simulink model "uz_endat_interface_2025b"  (R2025b)
settings: Solver=FixedStepDiscrete  StartTime=0.0  StopTime=1.3e-3  RelTol=1e-3
values from neighbouring files (symbols this model uses):
  binary_or_gray = false    [uz_endat_interface_init.m]
  bit_sum = endat_encoder_bit_width_multi_turn+endat_encoder_bit_width_single_turn+endat_encoder_number_of_CRC_bits    [uz_endat_interface_init.m]
  delay_first_clk_on_off = true    [uz_endat_interface_init.m]
  endat_clk_divider = 25    [uz_endat_interface_init.m]
  endat_encoder_bit_width_multi_turn = uint32(12)    [uz_endat_interface_init.m]
  endat_encoder_bit_width_single_turn = uint32(25)    [uz_endat_interface_init.m]
  endat_encoder_number_of_CRC_bits = uint32(0)    [uz_endat_interface_init.m]
  f_ADC = 20e3    (= 20000)    [uz_endat_interface_init.m]
  f_clock = 100e6    (= 100000000)    [uz_endat_interface_init.m]
  t_ADC = 1/f_ADC    (= 5e-05)    [uz_endat_interface_init.m]
  t_clock = 1/f_clock    (= 1e-08)    [uz_endat_interface_init.m]
undefined symbols (not defined in the file or in its folder): PLL
libraries: simulink x37, hdlsllib x32, simulink_extras x14, spsSampleandHoldLib x1
(part 2 of 3)

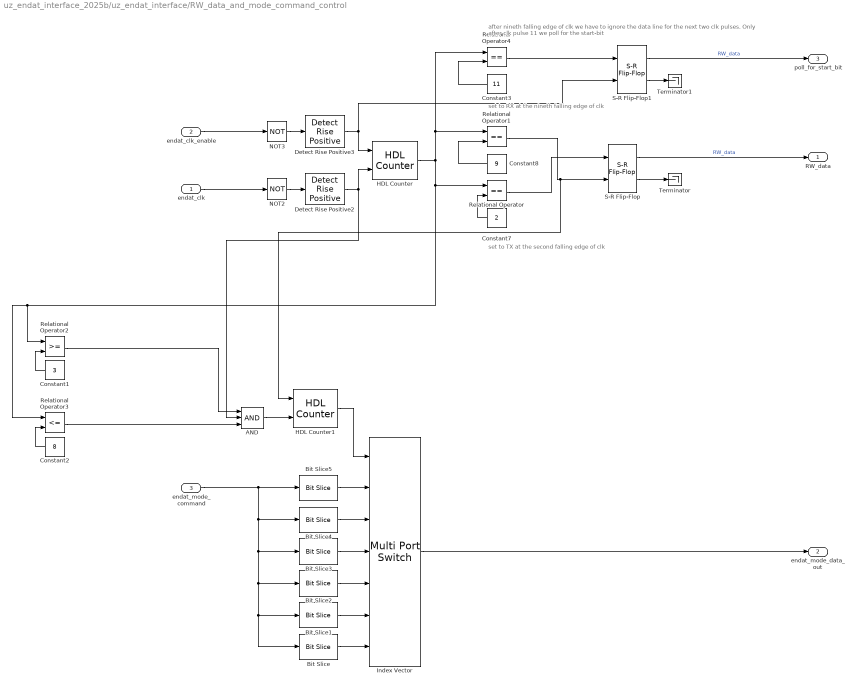
== system uz_endat_interface_2025b/uz_endat_interface/RW_data_and_mode_command_control ==
  note: set to TX at the second falling edge of clk
  note: set to RX at the nineth falling edge of clk
  note: after nineth falling edge of clk we have to ignore the data line for the next two clk pulses. Only after clk pulse 11 we poll for the start-bit
  endat_clk : Inport
  endat_clk_enable : Inport  Port=2
  endat_mode_command : Inport  Port=3
  AND : Logic  Inputs=3  IconShape=distinctive  AllPortsSameDT=off  OutDataTypeStr=boolean
  Bit Slice : hdlsllib/Logic and Bit Operations/Bit Slice  lidx=0  ridx=0
  Bit Slice1 : hdlsllib/Logic and Bit Operations/Bit Slice  lidx=1  ridx=1
  Bit Slice2 : hdlsllib/Logic and Bit Operations/Bit Slice  lidx=2  ridx=2
  Bit Slice3 : hdlsllib/Logic and Bit Operations/Bit Slice  lidx=3  ridx=3
  Bit Slice4 : hdlsllib/Logic and Bit Operations/Bit Slice  lidx=4  ridx=4
  Bit Slice5 : hdlsllib/Logic and Bit Operations/Bit Slice  lidx=5  ridx=5
  Constant1 : Constant  Value=3  OutDataTypeStr=uint8  SampleTime=-1
  Constant2 : Constant  Value=8  OutDataTypeStr=uint8  SampleTime=-1
  Constant3 : Constant  Value=11  OutDataTypeStr=uint8  SampleTime=-1
  Constant7 : Constant  Value=2  OutDataTypeStr=uint8  SampleTime=-1
  Constant8 : Constant  Value=9  OutDataTypeStr=uint8  SampleTime=-1
  Detect Rise Positive2 : simulink/Logic and Bit Operations/Detect Rise Positive  vinit=0  OutDataTypeStr=boolean
  Detect Rise Positive3 : simulink/Logic and Bit Operations/Detect Rise Positive  vinit=0  OutDataTypeStr=boolean
  HDL Counter : hdlsllib/Sources/HDL Counter  CountType=Free running  CountInit=0  CountStep=1  CountMax=25  CountFromType=Initial value  CountFrom=0  CountResetPort=on  CountLoadPort=off  CountEnbPort=on  CountDirPort=off  CountHitOutputPort=off  CountDataType=Unsigned  CountWordLen=8  CountFracLen=0  CountSampTime=1
  HDL Counter1 : hdlsllib/Sources/HDL Counter  CountType=Count limited  CountInit=0  CountStep=1  CountMax=5  CountFromType=Initial value  CountFrom=0  CountResetPort=on  CountLoadPort=off  CountEnbPort=on  CountDirPort=off  CountHitOutputPort=off  CountDataType=Unsigned  CountWordLen=8  CountFracLen=0  CountSampTime=1
  Index Vector : MultiPortSwitch  DataPortOrder=Zero-based contiguous  Inputs=6  zeroidx=on  SaturateOnIntegerOverflow=off  InputSameDT=off
  NOT2 : Logic  Operator=NOT  IconShape=distinctive  AllPortsSameDT=off  OutDataTypeStr=boolean
  NOT3 : Logic  Operator=NOT  IconShape=distinctive  AllPortsSameDT=off  OutDataTypeStr=boolean
  Relational Operator : RelationalOperator  Operator===  OutDataTypeStr=boolean  RndMeth=Simplest  InputSameDT=off
  Relational Operator1 : RelationalOperator  Operator===  OutDataTypeStr=boolean  RndMeth=Simplest  InputSameDT=off
  Relational Operator2 : RelationalOperator  OutDataTypeStr=boolean  RndMeth=Simplest  InputSameDT=off
  Relational Operator3 : RelationalOperator  Operator=<=  OutDataTypeStr=boolean  RndMeth=Simplest  InputSameDT=off
  Relational Operator4 : RelationalOperator  Operator===  OutDataTypeStr=boolean  RndMeth=Simplest  InputSameDT=off
  S-R Flip-Flop : simulink_extras/Flip Flops/S-R Flip-Flop  initial_condition=0
  S-R Flip-Flop1 : simulink_extras/Flip Flops/S-R Flip-Flop  initial_condition=0
  Terminator : Terminator
  Terminator1 : Terminator
  RW_data : Outport
  endat_mode_data_out : Outport  Port=2
  poll_for_start_bit : Outport  Port=3
  wires:
  Constant7/1 -> Relational Operator/2
  HDL Counter/1 -> Relational Operator2/1, Relational Operator3/1, Relational Operator/1, Relational Operator4/1, Relational Operator1/1
  endat_clk_enable/1 -> NOT3/1
  S-R Flip-Flop/2 -> Terminator/1
  Constant8/1 -> Relational Operator1/2
  NOT2/1 -> Detect Rise Positive2/1
  endat_clk/1 -> NOT2/1
  NOT3/1 -> Detect Rise Positive3/1
  S-R Flip-Flop/1 -> RW_data/1  "RW_data"
  Relational Operator/1 -> S-R Flip-Flop/1
  Detect Rise Positive3/1 -> HDL Counter/1, S-R Flip-Flop1/2
  Bit Slice/1 -> Index Vector/7
  Bit Slice3/1 -> Index Vector/4
  Bit Slice2/1 -> Index Vector/5
  Bit Slice1/1 -> Index Vector/6
  Bit Slice4/1 -> Index Vector/3
  Bit Slice5/1 -> Index Vector/2
  endat_mode_command/1 -> Bit Slice4/1, Bit Slice3/1, Bit Slice2/1, Bit Slice1/1, Bit Slice/1, Bit Slice5/1
  AND/1 -> HDL Counter1/2
  Constant1/1 -> Relational Operator2/2
  HDL Counter1/1 -> Index Vector/1
  Constant2/1 -> Relational Operator3/2
  Relational Operator1/1 -> HDL Counter1/1, S-R Flip-Flop/2
  Detect Rise Positive2/1 -> AND/2, HDL Counter/2
  Relational Operator2/1 -> AND/1
  Relational Operator3/1 -> AND/3
  Index Vector/1 -> endat_mode_data_out/1
  Constant3/1 -> Relational Operator4/2
  Relational Operator4/1 -> S-R Flip-Flop1/1
  S-R Flip-Flop1/1 -> poll_for_start_bit/1  "RW_data"
  S-R Flip-Flop1/2 -> Terminator1/1

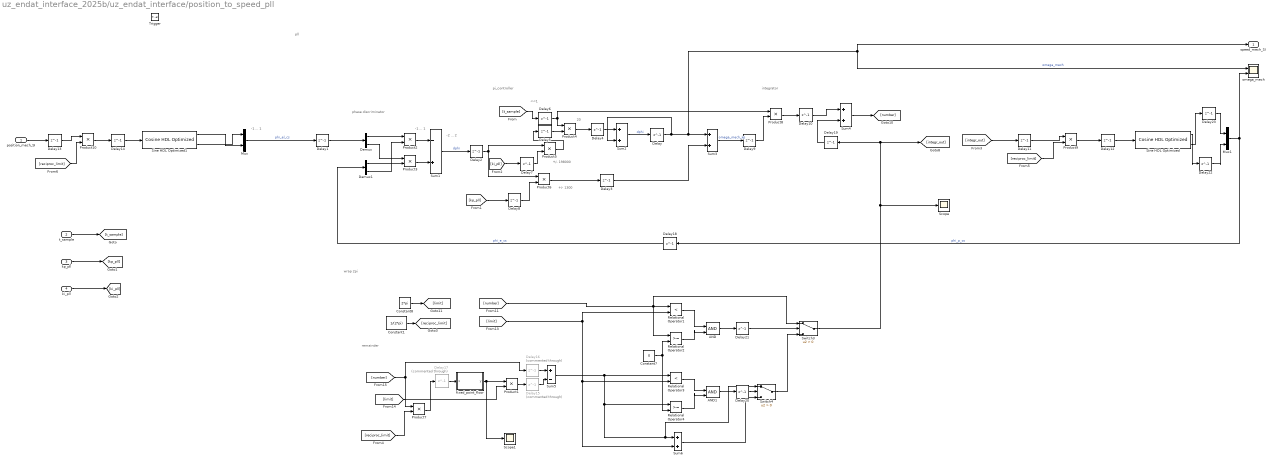
== system uz_endat_interface_2025b/uz_endat_interface/position_to_speed_pll ==
  note: remainder
  note: +/- 1300
  note: 20
  note: integrator
  note: -1 ... 1
  note: pll
  note: -1 ... 1
  note: phase discriminator
  note: <<1
  note: wrap 2pi
  note: -2 ... 2
  note: +/- 198000
  note: pi_controller
  position_mech_SI : Inport
  t_sample : Inport  Port=2
  kp_pll : Inport  Port=3
  ki_pll : Inport  Port=4
  Trigger : TriggerPort  VariantControl=(inherit)  InitialTriggerSignalState=zero
  AND : Logic  IconShape=distinctive  AllPortsSameDT=off  OutDataTypeStr=boolean
  AND1 : Logic  IconShape=distinctive  AllPortsSameDT=off  OutDataTypeStr=boolean
  Constant1 : Constant  Value=1/(2*pi)  OutDataTypeStr=fixdt(0,18,20)  SampleTime=-1
  Constant7 : Constant  Value=0  OutDataTypeStr=fixdt(0,27,24)  SampleTime=-1
  Constant8 : Constant  Value=2*pi  OutDataTypeStr=fixdt(0,18,15)  SampleTime=-1
  Delay{,19..23} (6 alike) : Delay  DelayLength=1
  Delay1 : Delay  DelayLength=1  InitialCondition=[1 0]
  Delay{2..14} (13 alike) : Delay  DelayLength=1  InitialCondition=0
  Delay15 : Delay  Commented=through  DelayLength=1  InitialCondition=0
  Delay16 : Delay  Commented=through  DelayLength=1  InitialCondition=0
  Delay17 : Delay  Commented=through  DelayLength=1  InitialCondition=0
  Delay18 : Delay  DelayLength=1  InitialCondition=[1 0]
  Demux : Demux  Outputs=2
  Demux1 : Demux  Outputs=2
  Mux : Mux  Inputs=2
  Mux1 : Mux  Inputs=2
  Product1 : Product  OutDataTypeStr=fixdt(1,27,23)
  Product10 : Product  OutDataTypeStr=fixdt(1,27,20)
  Product2 : Product  OutDataTypeStr=fixdt(1,27,25)
  Product3 : Product  OutDataTypeStr=fixdt(1,27,25)
  Product4 : Product  OutDataTypeStr=fixdt(1,27,20)
  Product5 : Product  OutDataTypeStr=fixdt(1,27,8)
  Product6 : Product  OutDataTypeStr=fixdt(1,27,14)
  Product7 : Product  OutDataTypeStr=fixdt(1,27,23)
  Product8 : Product  OutDataTypeStr=fixdt(1,27,26)
  Product9 : Product  OutDataTypeStr=fixdt(1,27,20)
  Relational Operator1 : RelationalOperator  Operator=<  OutDataTypeStr=boolean  RndMeth=Simplest  InputSameDT=off
  Relational Operator2 : RelationalOperator  OutDataTypeStr=boolean  RndMeth=Simplest  InputSameDT=off
  Relational Operator3 : RelationalOperator  Operator=<  OutDataTypeStr=boolean  RndMeth=Simplest  InputSameDT=off
  Relational Operator4 : RelationalOperator  OutDataTypeStr=boolean  RndMeth=Simplest  InputSameDT=off
  Scope : Scope
      settings: ActiveDisplayYMinimum=0.18141  ActiveDisplayYMaximum=6.96115  DataLoggingVariableName=ScopeData2
  Scope1 : Scope
      settings: ActiveDisplayYMinimum=-0.125  ActiveDisplayYMaximum=1.125  DataLoggingVariableName=ScopeData2
  Sine HDL Optimized : hdlsllib/Lookup Tables/Cosine HDL Optimized  OutputFormula=sin(2*pi*u) and cos(2*pi*u)  NumDataPoints=256  TableDataTypeStr=fixdt(0,26,20)  SimulateLUTROMDelay=off
      settings: LibrarySourceBlock=|
      | hdlsllib/Lookup
      | Tables/Sine
      | HDL Optimized
  Sine HDL Optimized1 : hdlsllib/Lookup Tables/Cosine HDL Optimized  OutputFormula=sin(2*pi*u) and cos(2*pi*u)  NumDataPoints=256  TableDataTypeStr=fixdt(0,26,20)  SimulateLUTROMDelay=off
      settings: LibrarySourceBlock=|
      | hdlsllib/Lookup
      | Tables/Sine
      | HDL Optimized
  Sum1 : Sum  Inputs=-+  AccumDataTypeStr=fixdt(1,27,24)
  Sum2 : Sum  OutDataTypeStr=fixdt(1,27,16)
  Sum3 : Sum  OutDataTypeStr=fixdt(1,27,14)
  Sum4 : Sum  OutDataTypeStr=fixdt(1,27,23)
  Sum5 : Sum  Inputs=+-  OutDataTypeStr=fixdt(1,27,23)
  Sum6 : Sum  OutDataTypeStr=fixdt(1,27,23)
  Switch3 : Switch  Criteria=u2 > Threshold  SaturateOnIntegerOverflow=off  InputSameDT=off
  Switch4 : Switch  Criteria=u2 > Threshold  SaturateOnIntegerOverflow=off  InputSameDT=off
  fixed_point_floor : MATLAB Function  TreatAsAtomicUnit=on
  omega_mech : Scope  NumInputPorts=2
      settings: ActiveDisplayYMinimum=-587.14492  ActiveDisplayYMaximum=357.65664
  speed_mech_SI : Outport  InitialOutput=[0]
  wires:
  Product2/1 -> Sum1/1
  Constant8/1 -> [limit]
  Delay19/1 -> Sum4/2
  Demux/1 -> Product2/1
  Mux1/1 -> omega_mech/2, Delay18/1  "phi_p_cs"
  [ki_pll] -> Delay7/1
  Sine HDL Optimized/2 -> Delay23/1
  Sum3/1 -> Delay9/1  "omega_mech_kp"
  Demux1/2 -> Product2/2
  Switch3/1 -> Scope/1, Delay19/1, [integr_out]
  Product3/1 -> Sum1/2
  Product4/1 -> Delay4/1
  Delay/1 -> speed_mech_SI/1, omega_mech/1, Sum3/1, Sum2/2  "omega_mech"
  Product8/1 -> Delay10/1
  [limit] -> Product1/2
  Switch4/1 -> Switch3/3
  [integr_out] -> Delay11/1
  Product1/1 -> Delay15/1
  Relational Operator3/1 -> AND1/1
  Product9/1 -> Delay12/1
  [number] -> Relational Operator2/1, Switch3/1, Relational Operator1/1
  Relational Operator2/1 -> AND/2
  Sum4/1 -> [number]
  Sum1/1 -> Delay2/1  "dphi"
  [limit] -> Relational Operator1/2, Sum6/2, Relational Operator3/2
  Product5/1 -> Delay5/1
  Product10/1 -> Delay14/1
  [number] -> Product7/1, Delay16/1
  Demux/2 -> Product3/1
  Delay6/1 -> Product4/1, Product8/1
  Demux1/1 -> Product3/2
  Delay18/1 -> Demux1/1  "phi_e_cs"
  Sine HDL Optimized/1 -> Delay22/1
  Mux/1 -> Delay1/1  "phi_el_cs"
  Relational Operator1/1 -> AND/1
  Product6/1 -> Delay3/1
  [kp_pll] -> Delay8/1
  AND/1 -> Delay21/1
  Sine HDL Optimized1/1 -> Mux/2
  Product7/1 -> Delay17/1
  Sum2/1 -> Delay/1  "dphi"
  Sum6/1 -> Switch4/3
  Sine HDL Optimized1/2 -> Mux/1
  Relational Operator4/1 -> AND1/2
  AND1/1 -> Delay20/1
  fixed_point_floor/1(y) -> Product1/1, Scope1/1
  position_mech_SI/1 -> Delay13/1
  Constant7/1 -> Relational Operator2/2, Relational Operator4/2
  t_sample/1 -> [t_sample]
  kp_pll/1 -> [kp_pll]
  ki_pll/1 -> [ki_pll]
  Delay1/1 -> Demux/1
  Delay2/1 -> Product5/1, Product6/1
  Delay3/1 -> Sum3/2
  Delay4/1 -> Sum2/1
  Delay5/1 -> Product4/2
  Delay7/1 -> Product5/2
  Delay8/1 -> Product6/2
  Delay9/1 -> Product8/2
  [t_sample] -> Delay6/1
  Delay10/1 -> Sum4/1
  Delay11/1 -> Product9/1
  Delay12/1 -> Sine HDL Optimized/1
  Delay13/1 -> Product10/1
  Delay14/1 -> Sine HDL Optimized1/1
  Delay15/1 -> Sum5/2
  Delay16/1 -> Sum5/1
  Delay17/1 -> fixed_point_floor/1(x)
  Sum5/1 -> Switch4/1, Sum6/1, Relational Operator4/1, Relational Operator3/1
  Constant1/1 -> [reciproc_limit]
  [reciproc_limit] -> Product7/2
  Delay20/1 -> Switch4/2
  Delay21/1 -> Switch3/2
  [reciproc_limit] -> Product9/2
  [reciproc_limit] -> Product10/2
  Delay22/1 -> Mux1/2
  Delay23/1 -> Mux1/1

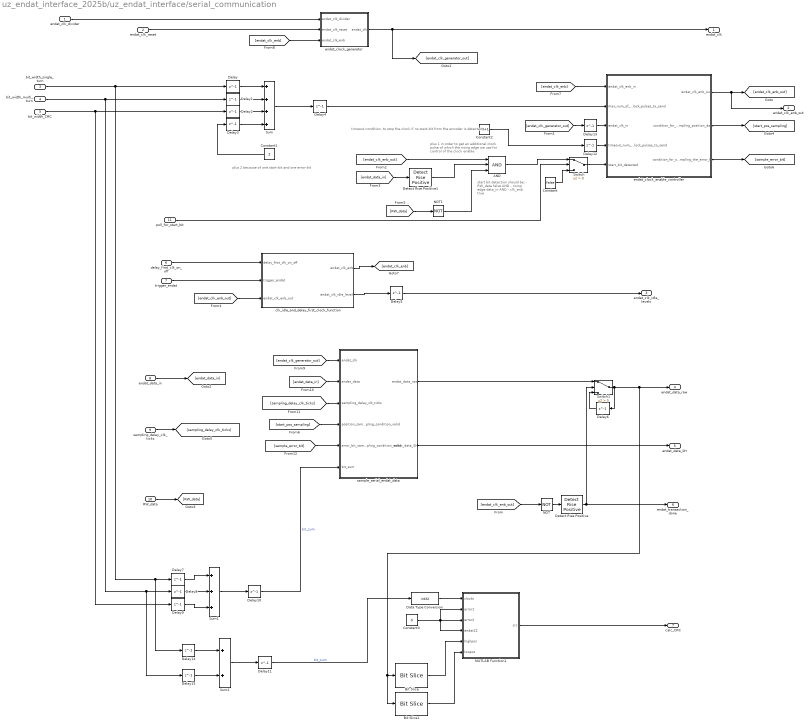
== system uz_endat_interface_2025b/uz_endat_interface/serial_communication ==
  note: plus 2 because of one start-bit and one error-bit
  note: timeout condition, to stop the clock if no start-bit from the encoder is detected
  note: plus 1 in order to get an additional clock pulse of which the rising edge we use for control of the clock enable
  note: start bit detection should be:
      | - RW_data false
      | AND
      | - rising edge data_in
      | AND
      | - clk_enb true
  endat_clk_divider : Inport
  endat_clk_reset : Inport  Port=2
  bit_width_single_turn : Inport  Port=3  OutDataTypeStr=uint32
  bit_width_multi_turn : Inport  Port=4  OutDataTypeStr=uint32
  bit_width_CRC : Inport  Port=5  OutDataTypeStr=uint32
  delay_first_clk_on_off : Inport  Port=6
  trigger_endat : Inport  Port=7
  endat_data_in : Inport  Port=8
  sampling_delay_clk_ticks : Inport  Port=9  OutDataTypeStr=uint32
  RW_data : Inport  Port=10
  poll_for_start_bit : Inport  Port=11
  AND : Logic  Inputs=3  IconShape=distinctive  AllPortsSameDT=off  OutDataTypeStr=boolean
  Bit Slice : hdlsllib/Logic and Bit Operations/Bit Slice  lidx=63  ridx=32
  Bit Slice1 : hdlsllib/Logic and Bit Operations/Bit Slice  lidx=31  ridx=0
  Constant : Constant  Value=false  SampleTime=-1
  Constant1 : Constant  Value=2  OutDataTypeStr=uint32  SampleTime=t_clock
  Constant2 : Constant  Value=70+1  OutDataTypeStr=uint32  SampleTime=t_clock
  Constant3 : Constant  Value=0  OutDataTypeStr=uint32  SampleTime=-1
  Data Type Conversion : DataTypeConversion  OutDataTypeStr=int32  SaturateOnIntegerOverflow=off  RndMeth=Floor
  Delay{,1..4,7..11,14..15} (12 alike) : Delay  DelayLength=1  InitialCondition=0
  Delay{5..6,12..13} (4 alike) : Delay  DelayLength=1
  Detect Rise Positive : simulink/Logic and Bit Operations/Detect Rise Positive  vinit=0  OutDataTypeStr=boolean
  Detect Rise Positive1 : simulink/Logic and Bit Operations/Detect Rise Positive  vinit=0  OutDataTypeStr=boolean
  MATLAB Function1 : MATLAB Function  TreatAsAtomicUnit=on
  NOT : Logic  Operator=NOT  IconShape=distinctive  AllPortsSameDT=off  OutDataTypeStr=boolean
  NOT1 : Logic  Operator=NOT  IconShape=distinctive  AllPortsSameDT=off  OutDataTypeStr=boolean
  Sum : Sum  Inputs=++++  OutDataTypeStr=uint32
  Sum1 : Sum  Inputs=+++  OutDataTypeStr=uint32
  Sum2 : Sum  OutDataTypeStr=uint32
  Switch : Switch  Criteria=u2 > Threshold  SaturateOnIntegerOverflow=off  InputSameDT=off
  Switch1 : Switch  Criteria=u2 > Threshold  SaturateOnIntegerOverflow=off  InputSameDT=off
  clk_idle_and_delay_first_clock_function : Subsystem
  endat_clock_enable_controller : Subsystem
  endat_clock_generator : Subsystem
  sample_serial_endat_data : Subsystem
  endat_clk : Outport
  endat_clk_enb_out : Outport  Port=2
  endat_clk_idle_levels : Outport  Port=3
  endat_data_raw : Outport  Port=4
  endat_data_SH : Outport  Port=5
  endat_transaction_done : Outport  Port=6
  calc_CRC : Outport  Port=7
  wires:
  Delay5/1 -> endat_clk_idle_levels/1
  [endat_clk_generator_out] -> sample_serial_endat_data/1(endat_clk)
  [endat_clk_enb] -> endat_clock_enable_controller/1(endat_clk_enb_in)
  endat_data_in/1 -> [endat_data_in]
  [endat_clk_generator_out] -> Delay13/1
  Detect Rise Positive/1 -> Switch1/2, endat_transaction_done/1
  Constant2/1 -> Delay12/1
  Delay12/1 -> endat_clock_enable_controller/4(timeout_num_of_clock_pulses_to_send)
  clk_idle_and_delay_first_clock_function/2(endat_clk_idle_levels) -> Delay5/1
  [endat_clk_enb_out] -> clk_idle_and_delay_first_clock_function/3(endat_clk_enb_out)
  endat_clock_enable_controller/1(endat_clk_enb_out) -> endat_clk_enb_out/1, [endat_clk_enb_out]
  Delay13/1 -> endat_clock_enable_controller/3(endat_clk_in)
  [endat_clk_enb] -> endat_clock_generator/3(endat_clk_enb)
  clk_idle_and_delay_first_clock_function/1(endat_clk_enb) -> [endat_clk_enb]
  sample_serial_endat_data/1(endat_data_raw) -> Switch1/1
  sample_serial_endat_data/2(endat_data_SH) -> endat_data_SH/1
  endat_clk_divider/1 -> endat_clock_generator/1(endat_clk_divider)
  endat_clk_reset/1 -> endat_clock_generator/2(endat_clk_reset)
  trigger_endat/1 -> clk_idle_and_delay_first_clock_function/2(trigger_endat)
  NOT/1 -> Detect Rise Positive/1
  [endat_clk_enb_out] -> NOT/1
  delay_first_clk_on_off/1 -> clk_idle_and_delay_first_clock_function/1(delay_first_clk_on_off)
  Constant1/1 -> Delay3/1
  [start_pos_sampling] -> sample_serial_endat_data/4(position_sampling_condition_valid)
  Sum/1 -> Delay4/1
  Switch/1 -> endat_clock_enable_controller/5(start_bit_detected)
  [endat_clk_enb_out] -> AND/1
  [endat_data_in] -> Detect Rise Positive1/1
  Detect Rise Positive1/1 -> AND/2
  RW_data/1 -> [RW_data]
  [RW_data] -> NOT1/1
  endat_clock_generator/1(endat_clk) -> endat_clk/1, [endat_clk_generator_out]
  NOT1/1 -> AND/3
  endat_clock_enable_controller/2(condition_for_start_sampling_position_data) -> [start_pos_sampling]
  [endat_data_in] -> sample_serial_endat_data/2(endat_data)
  sampling_delay_clk_ticks/1 -> [sampling_delay_clk_ticks]
  [sampling_delay_clk_ticks] -> sample_serial_endat_data/3(sampling_delay_clk_ticks)
  endat_clock_enable_controller/3(condition_for_sampling_the_error_bit) -> [sample_error_bit]
  [sample_error_bit] -> sample_serial_endat_data/5(error_bit_sampling_condition_valid)
  Delay/1 -> Sum/1
  Delay1/1 -> Sum/2
  Delay2/1 -> Sum/3
  Delay3/1 -> Sum/4
  Delay4/1 -> endat_clock_enable_controller/2(max_num_of_clock_pulses_to_send)
  AND/1 -> Switch/1
  poll_for_start_bit/1 -> Switch/2
  Constant/1 -> Switch/3
  Delay6/1 -> Switch1/3
  Switch1/1 -> Delay6/1, Bit Slice1/1, Bit Slice/1, endat_data_raw/1
  Delay7/1 -> Sum1/1
  Delay8/1 -> Sum1/2
  Sum1/1 -> Delay10/1
  bit_width_single_turn/1 -> Delay14/1, Delay7/1, Delay/1
  bit_width_CRC/1 -> Delay9/1, Delay2/1
  Delay9/1 -> Sum1/3
  bit_width_multi_turn/1 -> Delay15/1, Delay8/1, Delay1/1
  Delay10/1 -> sample_serial_endat_data/6(bit_sum)  "bit_sum"
  Delay15/1 -> Sum2/2
  Sum2/1 -> Delay11/1
  Delay14/1 -> Sum2/1
  Delay11/1 -> Data Type Conversion/1  "bit_sum"
  Constant3/1 -> MATLAB Function1/4(endat22), MATLAB Function1/3(error2), MATLAB Function1/2(error1)
  Bit Slice/1 -> MATLAB Function1/5(highpos)
  Bit Slice1/1 -> MATLAB Function1/6(lowpos)
  MATLAB Function1/1(crc) -> calc_CRC/1
  Data Type Conversion/1 -> MATLAB Function1/1(clocks)

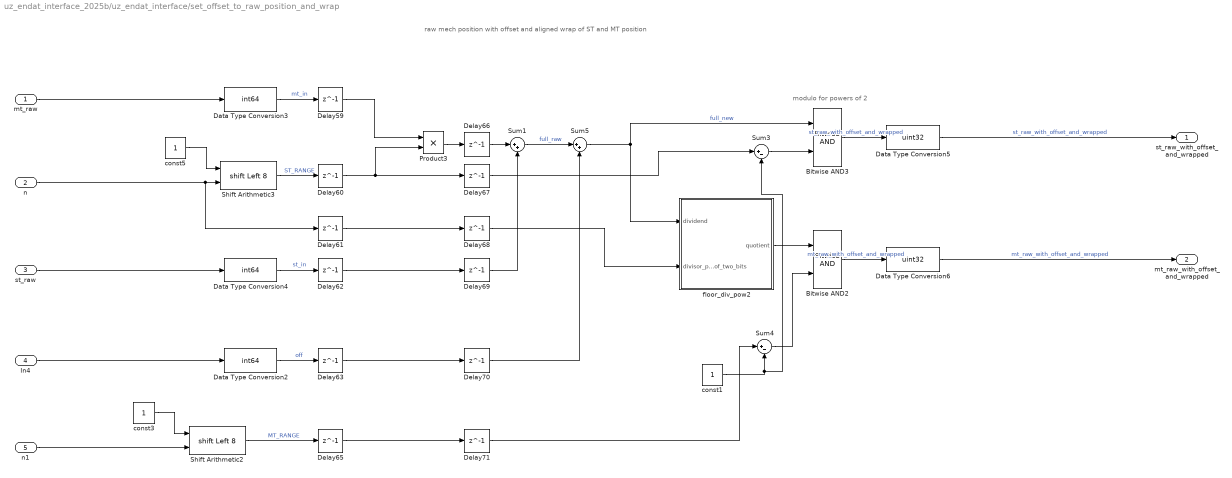
== system uz_endat_interface_2025b/uz_endat_interface/set_offset_to_raw_position_and_wrap ==
  note: raw mech position with offset and aligned wrap of ST and MT position
  note: modulo for powers of 2
  mt_raw : Inport
  n : Inport  Port=2
  st_raw : Inport  Port=3
  In4 : Inport  Port=4
  n1 : Inport  Port=5
  Bitwise AND2 : simulink/Logic and Bit Operations/Bitwise Operator  logicop=AND  UseBitMask=off  NumInputPorts=2  BitMask=bin2dec('11011001')  BitMaskRealWorld=Stored Integer
      settings: LibrarySourceBlock=|
      | simulink/Quick Insert/Logic and Bit
      | Operations/Bitwise AND
  Bitwise AND3 : simulink/Logic and Bit Operations/Bitwise Operator  logicop=AND  UseBitMask=off  NumInputPorts=2  BitMask=bin2dec('11011001')  BitMaskRealWorld=Stored Integer
      settings: LibrarySourceBlock=|
      | simulink/Quick Insert/Logic and Bit
      | Operations/Bitwise AND
  Data Type Conversion2 : DataTypeConversion  OutDataTypeStr=int64  SaturateOnIntegerOverflow=off  RndMeth=Floor
  Data Type Conversion3 : DataTypeConversion  OutDataTypeStr=int64  SaturateOnIntegerOverflow=off  RndMeth=Floor
  Data Type Conversion4 : DataTypeConversion  OutDataTypeStr=int64  SaturateOnIntegerOverflow=off  RndMeth=Floor
  Data Type Conversion5 : DataTypeConversion  OutDataTypeStr=uint32  SaturateOnIntegerOverflow=off  RndMeth=Floor
  Data Type Conversion6 : DataTypeConversion  OutDataTypeStr=uint32  SaturateOnIntegerOverflow=off  RndMeth=Floor
  Delay{59..63,65..71} (12 alike) : Delay  DelayLength=1  InitialCondition=0
  Product3 : Product  OutDataTypeStr=int64
  Shift Arithmetic2 : ArithShift  BitShiftNumberSource=Input port  BitShiftNumber=8  BitShiftDirection=Left
      settings: InputPortMap=u0,p1
  Shift Arithmetic3 : ArithShift  BitShiftNumberSource=Input port  BitShiftNumber=8  BitShiftDirection=Left
      settings: InputPortMap=u0,p1
  Sum1 : Sum  Inputs=|++  OutDataTypeStr=int64
  Sum3 : Sum  Inputs=|+-  OutDataTypeStr=int64
  Sum4 : Sum  Inputs=|+-  OutDataTypeStr=int64
  Sum5 : Sum  Inputs=|++  OutDataTypeStr=int64
  const1 : Constant  OutDataTypeStr=int64  SampleTime=t_clock
  const3 : Constant  OutDataTypeStr=int64  SampleTime=t_clock
  const5 : Constant  OutDataTypeStr=int64  SampleTime=t_clock
  floor_div_pow2 : Subsystem
  st_raw_with_offset_and_wrapped : Outport
  mt_raw_with_offset_and_wrapped : Outport  Port=2
  wires:
  mt_raw/1 -> Data Type Conversion3/1
  Delay62/1 -> Delay69/1
  Delay60/1 -> Product3/2, Delay67/1
  Data Type Conversion2/1 -> Delay63/1  "off"
  Data Type Conversion4/1 -> Delay62/1  "st_in"
  Delay70/1 -> Sum5/2
  Data Type Conversion3/1 -> Delay59/1  "mt_in"
  const1/1 -> Sum3/2, Sum4/2
  Delay68/1 -> floor_div_pow2/2(divisor_power_of_two_bits)
  Sum1/1 -> Sum5/1  "full_raw"
  Sum5/1 -> Bitwise AND3/1, floor_div_pow2/1(dividend)  "full_new"
  Product3/1 -> Delay66/1
  n/1 -> Delay61/1, Shift Arithmetic3/2
  Shift Arithmetic2/1 -> Delay65/1  "MT_RANGE"
  floor_div_pow2/1(quotient) -> Bitwise AND2/1
  Delay63/1 -> Delay70/1
  Bitwise AND3/1 -> Data Type Conversion5/1  "st_raw_with_offset_and_wrapped"
  Delay66/1 -> Sum1/1
  const5/1 -> Shift Arithmetic3/1
  const3/1 -> Shift Arithmetic2/1
  Bitwise AND2/1 -> Data Type Conversion6/1  "mt_raw_with_offset_and_wrapped"
  Delay71/1 -> Sum4/1
  Sum4/1 -> Bitwise AND2/2
  Shift Arithmetic3/1 -> Delay60/1  "ST_RANGE"
  st_raw/1 -> Data Type Conversion4/1
  Sum3/1 -> Bitwise AND3/2
  Delay61/1 -> Delay68/1
  Data Type Conversion6/1 -> mt_raw_with_offset_and_wrapped/1  "mt_raw_with_offset_and_wrapped"
  Delay65/1 -> Delay71/1
  Delay69/1 -> Sum1/2
  Delay67/1 -> Sum3/1
  Delay59/1 -> Product3/1
  In4/1 -> Data Type Conversion2/1
  n1/1 -> Shift Arithmetic2/2
  Data Type Conversion5/1 -> st_raw_with_offset_and_wrapped/1  "st_raw_with_offset_and_wrapped"

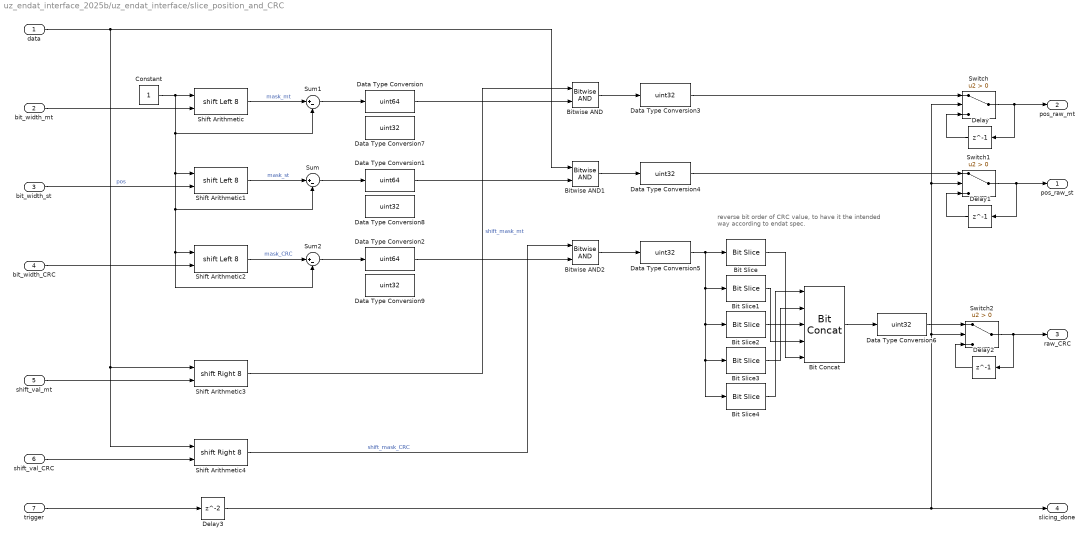
== system uz_endat_interface_2025b/uz_endat_interface/slice_position_and_CRC ==
  note: reverse bit order of CRC value, to have it
      | the intended way according to endat spec.
  data : Inport
  bit_width_mt : Inport  Port=2
  bit_width_st : Inport  Port=3
  bit_width_CRC : Inport  Port=4
  shift_val_mt : Inport  Port=5
  shift_val_CRC : Inport  Port=6
  trigger : Inport  Port=7
  Bit Concat : hdlsllib/Logic and Bit Operations/Bit Concat  numInputs=5
  Bit Slice : hdlsllib/Logic and Bit Operations/Bit Slice  lidx=4  ridx=4
  Bit Slice1 : hdlsllib/Logic and Bit Operations/Bit Slice  lidx=3  ridx=3
  Bit Slice2 : hdlsllib/Logic and Bit Operations/Bit Slice  lidx=2  ridx=2
  Bit Slice3 : hdlsllib/Logic and Bit Operations/Bit Slice  lidx=1  ridx=1
  Bit Slice4 : hdlsllib/Logic and Bit Operations/Bit Slice  lidx=0  ridx=0
  Bitwise AND : simulink/Logic and Bit Operations/Bitwise Operator  logicop=AND  UseBitMask=off  NumInputPorts=2  BitMask=bin2dec('11011001')  BitMaskRealWorld=Stored Integer
      settings: LibrarySourceBlock=|
      | simulink/Quick Insert/Logic and Bit
      | Operations/Bitwise AND
  Bitwise AND1 : simulink/Logic and Bit Operations/Bitwise Operator  logicop=AND  UseBitMask=off  NumInputPorts=2  BitMask=bin2dec('11011001')  BitMaskRealWorld=Stored Integer
      settings: LibrarySourceBlock=|
      | simulink/Quick Insert/Logic and Bit
      | Operations/Bitwise AND
  Bitwise AND2 : simulink/Logic and Bit Operations/Bitwise Operator  logicop=AND  UseBitMask=off  NumInputPorts=2  BitMask=bin2dec('11011001')  BitMaskRealWorld=Stored Integer
      settings: LibrarySourceBlock=|
      | simulink/Quick Insert/Logic and Bit
      | Operations/Bitwise AND
  Constant : Constant  OutDataTypeStr=uint32  SampleTime=t_clock
  Data Type Conversion : DataTypeConversion  OutDataTypeStr=uint64  SaturateOnIntegerOverflow=off  RndMeth=Floor
  Data Type Conversion1 : DataTypeConversion  OutDataTypeStr=uint64  SaturateOnIntegerOverflow=off  RndMeth=Floor
  Data Type Conversion2 : DataTypeConversion  OutDataTypeStr=uint64  SaturateOnIntegerOverflow=off  RndMeth=Floor
  Data Type Conversion{3..9} (7 alike) : DataTypeConversion  OutDataTypeStr=uint32  SaturateOnIntegerOverflow=off  RndMeth=Floor
  Delay : Delay  DelayLength=1
  Delay1 : Delay  DelayLength=1
  Delay2 : Delay  DelayLength=1
  Delay3 : Delay
  Shift Arithmetic : ArithShift  BitShiftNumberSource=Input port  BitShiftNumber=8  BitShiftDirection=Left
      settings: InputPortMap=u0,p1
  Shift Arithmetic1 : ArithShift  BitShiftNumberSource=Input port  BitShiftNumber=8  BitShiftDirection=Left
      settings: InputPortMap=u0,p1
  Shift Arithmetic2 : ArithShift  BitShiftNumberSource=Input port  BitShiftNumber=8  BitShiftDirection=Left
      settings: InputPortMap=u0,p1
  Shift Arithmetic3 : ArithShift  BitShiftNumberSource=Input port  BitShiftNumber=8  BitShiftDirection=Right
      settings: InputPortMap=u0,p1
  Shift Arithmetic4 : ArithShift  BitShiftNumberSource=Input port  BitShiftNumber=8  BitShiftDirection=Right
      settings: InputPortMap=u0,p1
  Sum : Sum  Inputs=|+-  OutDataTypeStr=uint32
  Sum1 : Sum  Inputs=|+-  OutDataTypeStr=uint32
  Sum2 : Sum  Inputs=|+-  OutDataTypeStr=uint32
  Switch : Switch  Criteria=u2 > Threshold  SaturateOnIntegerOverflow=off  InputSameDT=off
  Switch1 : Switch  Criteria=u2 > Threshold  SaturateOnIntegerOverflow=off  InputSameDT=off
  Switch2 : Switch  Criteria=u2 > Threshold  SaturateOnIntegerOverflow=off  InputSameDT=off
  pos_raw_st : Outport
  pos_raw_mt : Outport  Port=2
  raw_CRC : Outport  Port=3
  slicing_done : Outport  Port=4
  wires:
  Constant/1 -> Shift Arithmetic/1, Sum1/2, Shift Arithmetic1/1, Shift Arithmetic2/1, Sum2/2, Sum/2
  Shift Arithmetic1/1 -> Sum/1  "mask_st"
  bit_width_st/1 -> Shift Arithmetic1/2  "pos"
  Sum/1 -> Data Type Conversion1/1
  bit_width_mt/1 -> Shift Arithmetic/2
  bit_width_CRC/1 -> Shift Arithmetic2/2
  Shift Arithmetic/1 -> Sum1/1  "mask_mt"
  Shift Arithmetic2/1 -> Sum2/1  "mask_CRC"
  Sum1/1 -> Data Type Conversion/1
  Sum2/1 -> Data Type Conversion2/1
  Bitwise AND2/1 -> Data Type Conversion5/1
  data/1 -> Bitwise AND1/1, Shift Arithmetic4/1, Shift Arithmetic3/1
  Bitwise AND/1 -> Data Type Conversion3/1
  Bitwise AND1/1 -> Data Type Conversion4/1
  shift_val_mt/1 -> Shift Arithmetic3/2
  shift_val_CRC/1 -> Shift Arithmetic4/2
  Shift Arithmetic3/1 -> Bitwise AND/1  "shift_mask_mt"
  Data Type Conversion1/1 -> Bitwise AND1/2
  Data Type Conversion/1 -> Bitwise AND/2
  Data Type Conversion2/1 -> Bitwise AND2/2
  Shift Arithmetic4/1 -> Bitwise AND2/1  "shift_mask_CRC"
  Data Type Conversion3/1 -> Switch/1
  Data Type Conversion4/1 -> Switch1/1
  Data Type Conversion5/1 -> Bit Slice4/1, Bit Slice3/1, Bit Slice2/1, Bit Slice1/1, Bit Slice/1
  Switch/1 -> Delay/1, pos_raw_mt/1
  Switch1/1 -> Delay1/1, pos_raw_st/1
  Switch2/1 -> Delay2/1, raw_CRC/1
  Delay2/1 -> Switch2/3
  Delay1/1 -> Switch1/3
  Delay/1 -> Switch/3
  trigger/1 -> Delay3/1
  Delay3/1 -> slicing_done/1, Switch1/2, Switch/2, Switch2/2
  Bit Slice2/1 -> Bit Concat/3
  Bit Slice/1 -> Bit Concat/5
  Bit Slice4/1 -> Bit Concat/1
  Bit Slice1/1 -> Bit Concat/4
  Bit Slice3/1 -> Bit Concat/2
  Bit Concat/1 -> Data Type Conversion6/1
  Data Type Conversion6/1 -> Switch2/1

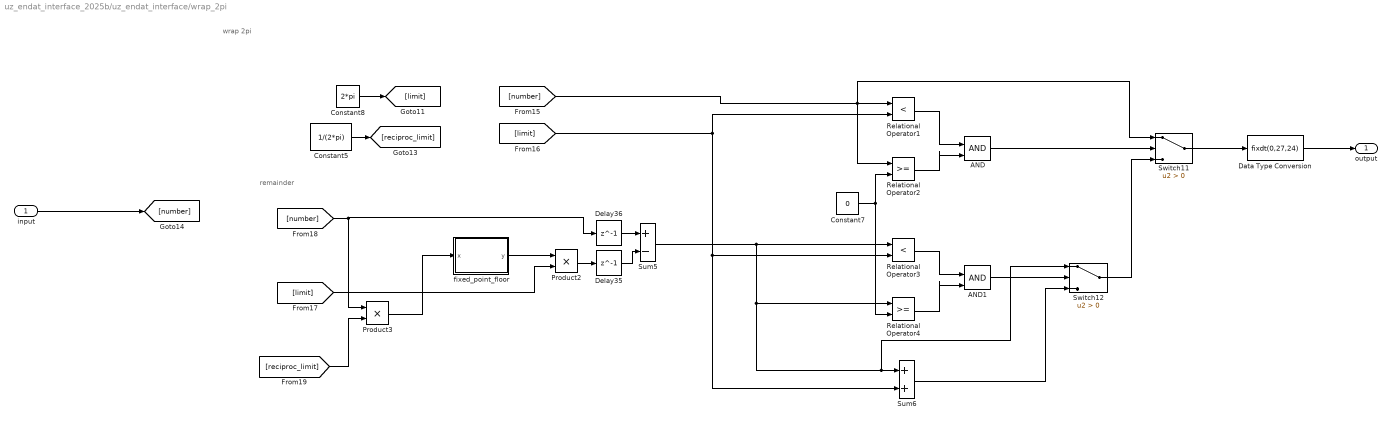
== system uz_endat_interface_2025b/uz_endat_interface/wrap_2pi ==
  note: wrap 2pi
  note: remainder
  input : Inport
  AND : Logic  IconShape=distinctive  AllPortsSameDT=off  OutDataTypeStr=boolean
  AND1 : Logic  IconShape=distinctive  AllPortsSameDT=off  OutDataTypeStr=boolean
  Constant5 : Constant  Value=1/(2*pi)  OutDataTypeStr=fixdt(0,18,20)  SampleTime=-1
  Constant7 : Constant  Value=0  OutDataTypeStr=fixdt(0,27,24)  SampleTime=-1
  Constant8 : Constant  Value=2*pi  OutDataTypeStr=fixdt(0,18,15)  SampleTime=-1
  Data Type Conversion : DataTypeConversion  OutDataTypeStr=fixdt(0,27,24)  SaturateOnIntegerOverflow=off  RndMeth=Floor
  Delay35 : Delay  DelayLength=1  InitialCondition=0
  Delay36 : Delay  DelayLength=1  InitialCondition=0
  Product2 : Product  OutDataTypeStr=fixdt(0,27,24)
  Product3 : Product  OutDataTypeStr=fixdt(0,27,24)
  Relational Operator1 : RelationalOperator  Operator=<  OutDataTypeStr=boolean  RndMeth=Simplest  InputSameDT=off
  Relational Operator2 : RelationalOperator  OutDataTypeStr=boolean  RndMeth=Simplest  InputSameDT=off
  Relational Operator3 : RelationalOperator  Operator=<  OutDataTypeStr=boolean  RndMeth=Simplest  InputSameDT=off
  Relational Operator4 : RelationalOperator  OutDataTypeStr=boolean  RndMeth=Simplest  InputSameDT=off
  Sum5 : Sum  Inputs=+-  OutDataTypeStr=fixdt(0,27,24)
  Sum6 : Sum  OutDataTypeStr=fixdt(0,27,24)
  Switch11 : Switch  Criteria=u2 > Threshold  SaturateOnIntegerOverflow=off  InputSameDT=off
  Switch12 : Switch  Criteria=u2 > Threshold  SaturateOnIntegerOverflow=off  InputSameDT=off
  fixed_point_floor : MATLAB Function  TreatAsAtomicUnit=on
  output : Outport
  wires:
  [number] -> Relational Operator2/1, Switch11/1, Relational Operator1/1
  Product2/1 -> Delay35/1
  [number] -> Delay36/1, Product3/1
  [reciproc_limit] -> Product3/2
  Delay35/1 -> Sum5/2
  Switch11/1 -> Data Type Conversion/1
  Relational Operator2/1 -> AND/2
  AND/1 -> Switch11/2
  Sum5/1 -> Switch12/1, Sum6/1, Relational Operator4/1, Relational Operator3/1
  Relational Operator1/1 -> AND/1
  [limit] -> Relational Operator1/2, Sum6/2, Relational Operator3/2
  Sum6/1 -> Switch12/3
  Delay36/1 -> Sum5/1
  Constant7/1 -> Relational Operator2/2, Relational Operator4/2
  Constant5/1 -> [reciproc_limit]
  Relational Operator4/1 -> AND1/2
  fixed_point_floor/1(y) -> Product2/1
  Product3/1 -> fixed_point_floor/1(x)
  AND1/1 -> Switch12/2
  [limit] -> Product2/2
  input/1 -> [number]
  Relational Operator3/1 -> AND1/1
  Switch12/1 -> Switch11/3
  Constant8/1 -> [limit]
  Data Type Conversion/1 -> output/1

== system uz_endat_interface_2025b/uz_endat_interface/Gray_code_to_binary/gray_to_bin ==
  gray : Inport
  enb : Inport  Port=2
  Bitwise OR1 : simulink/Logic and Bit Operations/Bitwise Operator  logicop=XOR  UseBitMask=off  NumInputPorts=2  BitMask=bin2dec('11011001')  BitMaskRealWorld=Stored Integer
      settings: LibrarySourceBlock=|
      | simulink/Quick Insert/Logic and Bit
      | Operations/Bitwise OR
  Constant4 : Constant  Value=63  OutMin=0  OutMax=63  OutDataTypeStr=fixdt(0,6)  SampleTime=t_clock
  Delay : Delay  DelayLength=1
  Delay2 : Delay  DelayLength=1
  Detect Rise Positive : simulink/Logic and Bit Operations/Detect Rise Positive  vinit=0  OutDataTypeStr=boolean
  Detect Rise Positive1 : simulink/Logic and Bit Operations/Detect Rise Positive  vinit=0  OutDataTypeStr=boolean
  HDL Counter : hdlsllib/Sources/HDL Counter  CountType=Count limited  CountInit=0  CountStep=1  CountMax=63  CountFromType=Initial value  CountFrom=0  CountResetPort=on  CountLoadPort=off  CountEnbPort=on  CountDirPort=off  CountHitOutputPort=off  CountDataType=Unsigned  CountWordLen=6  CountFracLen=0  CountSampTime=t_clock
  OR : Logic  Operator=OR  IconShape=distinctive  AllPortsSameDT=off  OutDataTypeStr=boolean
  Relational Operator2 : RelationalOperator  Operator===  OutDataTypeStr=boolean  RndMeth=Simplest  InputSameDT=off
  S-R Flip-Flop : simulink_extras/Flip Flops/S-R Flip-Flop  initial_condition=0
  Shift Arithmetic : ArithShift  BitShiftNumberSource=Input port  BitShiftNumber=8  BitShiftDirection=Right
      settings: InputPortMap=u0,p1
  Switch : Switch  Criteria=u2 > Threshold  SaturateOnIntegerOverflow=off  InputSameDT=off
  Switch3 : Switch  Criteria=u2 > Threshold  SaturateOnIntegerOverflow=off  InputSameDT=off
  binary_out : Outport
  wires:
  gray/1 -> Shift Arithmetic/1, Switch/1
  HDL Counter/1 -> Relational Operator2/1, Shift Arithmetic/2  "count"
  Switch3/1 -> binary_out/1, Delay2/1
  Constant4/1 -> Relational Operator2/2
  Delay2/1 -> Switch3/3
  Shift Arithmetic/1 -> Bitwise OR1/2  "shift_val"
  Relational Operator2/1 -> Detect Rise Positive/1
  enb/1 -> S-R Flip-Flop/1, OR/1, Detect Rise Positive1/1
  S-R Flip-Flop/1 -> HDL Counter/2
  Detect Rise Positive/1 -> Switch3/2, S-R Flip-Flop/2
  OR/1 -> HDL Counter/1
  S-R Flip-Flop/2 -> OR/2
  Detect Rise Positive1/1 -> Switch/2
  Switch/1 -> Bitwise OR1/1
  Bitwise OR1/1 -> Switch3/1, Delay/1  "binary_tmp"
  Delay/1 -> Switch/3

== system uz_endat_interface_2025b/uz_endat_interface/serial_communication/clk_idle_and_delay_first_clock_function ==
  note: 194 equals 2.0µs
  note: set idle level of clk to high (one),
      | and pull low when trigger_endat_read
      | is triggered
  delay_first_clk_on_off : Inport
  trigger_endat : Inport  Port=2
  endat_clk_enb_out : Inport  Port=3
  Constant4 : Constant  Value=0  OutDataTypeStr=boolean  SampleTime=t_clock
  Constant5 : Constant  OutDataTypeStr=boolean  SampleTime=t_clock
  Delay : Delay  DelayLength=194
  Delay1 : Delay  DelayLength=1
  Detect Rise Positive2 : simulink/Logic and Bit Operations/Detect Rise Positive  vinit=0  OutDataTypeStr=boolean
  NOT : Logic  Operator=NOT  IconShape=distinctive  AllPortsSameDT=off  OutDataTypeStr=boolean
  S-R Flip-Flop : simulink_extras/Flip Flops/S-R Flip-Flop  initial_condition=0
  Switch : Switch  Criteria=u2 > Threshold  SaturateOnIntegerOverflow=off  InputSameDT=off
  Switch3 : Switch  Criteria=u2 > Threshold  SaturateOnIntegerOverflow=off  InputSameDT=off
  Switch4 : Switch  Criteria=u2 > Threshold  SaturateOnIntegerOverflow=off  InputSameDT=off
  Terminator : Terminator
  endat_clk_enb : Outport
  endat_clk_idle_levels : Outport  Port=2
  wires:
  S-R Flip-Flop/2 -> Terminator/1
  Constant5/1 -> Switch/3
  Constant4/1 -> Switch/1
  NOT/1 -> Detect Rise Positive2/1
  Detect Rise Positive2/1 -> S-R Flip-Flop/2
  endat_clk_enb_out/1 -> NOT/1
  Switch/1 -> endat_clk_idle_levels/1
  trigger_endat/1 -> S-R Flip-Flop/1
  Delay/1 -> Switch4/1
  delay_first_clk_on_off/1 -> Switch3/2
  S-R Flip-Flop/1 -> Switch/2, Delay/1, Delay1/1
  Switch4/1 -> Switch3/1
  Delay1/1 -> Switch3/3, Switch4/3, Switch4/2
  Switch3/1 -> endat_clk_enb/1

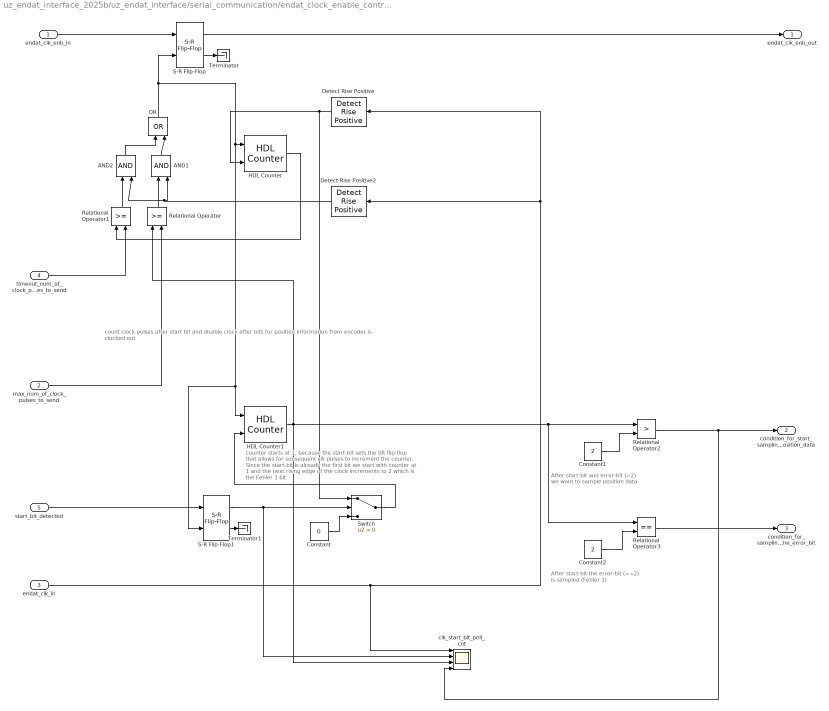
== system uz_endat_interface_2025b/uz_endat_interface/serial_communication/endat_clock_enable_controller ==
  note: counter starts at 1, because the start-bit sets the SR flip-flop that allows for subsequent clk pulses to increment the counter. Since the start-bit is already the first bit we start with counter at 1 and the next rising edge of the clock increments to 2 which is the Fehler 1 bit
  note: After start-bit and error-bit (=2)
      | we want to sample position data
  note: count clock pulses after start bit and disable clock after bits for position information from encoder is clocked out
  note: After start-bit the error-bit (==2)
      | is sampled (Fehler 1)
  endat_clk_enb_in : Inport
  max_num_of_clock_pulses_to_send : Inport  Port=2
  endat_clk_in : Inport  Port=3
  timeout_num_of_clock_pulses_to_send : Inport  Port=4
  start_bit_detected : Inport  Port=5
  AND1 : Logic  IconShape=distinctive  AllPortsSameDT=off  OutDataTypeStr=boolean
  AND2 : Logic  IconShape=distinctive  AllPortsSameDT=off  OutDataTypeStr=boolean
  Constant : Constant  Value=0  OutDataTypeStr=boolean  SampleTime=-1
  Constant1 : Constant  Value=2  OutDataTypeStr=uint8  SampleTime=-1
  Constant2 : Constant  Value=2  OutDataTypeStr=uint8  SampleTime=-1
  Detect Rise Positive : simulink/Logic and Bit Operations/Detect Rise Positive  vinit=0  OutDataTypeStr=boolean
  Detect Rise Positive2 : simulink/Logic and Bit Operations/Detect Rise Positive  vinit=0  OutDataTypeStr=boolean
  HDL Counter : hdlsllib/Sources/HDL Counter  CountType=Free running  CountInit=0  CountStep=1  CountMax=25  CountFromType=Initial value  CountFrom=0  CountResetPort=on  CountLoadPort=off  CountEnbPort=on  CountDirPort=off  CountHitOutputPort=off  CountDataType=Unsigned  CountWordLen=8  CountFracLen=0  CountSampTime=1
  HDL Counter1 : hdlsllib/Sources/HDL Counter  CountType=Free running  CountInit=1  CountStep=1  CountMax=25  CountFromType=Initial value  CountFrom=1  CountResetPort=on  CountLoadPort=off  CountEnbPort=on  CountDirPort=off  CountHitOutputPort=off  CountDataType=Unsigned  CountWordLen=8  CountFracLen=0  CountSampTime=1
  OR : Logic  Operator=OR  IconShape=distinctive  AllPortsSameDT=off  OutDataTypeStr=boolean
  Relational Operator : RelationalOperator  OutDataTypeStr=boolean  RndMeth=Simplest  InputSameDT=off
  Relational Operator1 : RelationalOperator  OutDataTypeStr=boolean  RndMeth=Simplest  InputSameDT=off
  Relational Operator2 : RelationalOperator  Operator=>  OutDataTypeStr=boolean  RndMeth=Simplest  InputSameDT=off
  Relational Operator3 : RelationalOperator  Operator===  OutDataTypeStr=boolean  RndMeth=Simplest  InputSameDT=off
  S-R Flip-Flop : simulink_extras/Flip Flops/S-R Flip-Flop  initial_condition=0
  S-R Flip-Flop1 : simulink_extras/Flip Flops/S-R Flip-Flop  initial_condition=0
  Switch : Switch  Criteria=u2 > Threshold  SaturateOnIntegerOverflow=off  InputSameDT=off
  Terminator : Terminator
  Terminator1 : Terminator
  clk_start_bit_poll_cnt : Scope  NumInputPorts=4
      settings: ActiveDisplayYMinimum=-0.125  ActiveDisplayYMaximum=1.125  DataLoggingVariableName=ScopeData3
  endat_clk_enb_out : Outport
  condition_for_start_sampling_position_data : Outport  Port=2
  condition_for_sampling_the_error_bit : Outport  Port=3
  wires:
  HDL Counter/1 -> Relational Operator1/1
  max_num_of_clock_pulses_to_send/1 -> Relational Operator/2
  S-R Flip-Flop/2 -> Terminator/1
  Relational Operator/1 -> AND1/1
  Detect Rise Positive/1 -> Switch/1, HDL Counter/2
  endat_clk_in/1 -> clk_start_bit_poll_cnt/1, Detect Rise Positive/1, Detect Rise Positive2/1
  S-R Flip-Flop/1 -> endat_clk_enb_out/1
  Detect Rise Positive2/1 -> AND2/2, AND1/2
  endat_clk_enb_in/1 -> S-R Flip-Flop/1
  AND1/1 -> OR/2
  Relational Operator1/1 -> AND2/1
  timeout_num_of_clock_pulses_to_send/1 -> Relational Operator1/2
  AND2/1 -> OR/1
  HDL Counter1/1 -> clk_start_bit_poll_cnt/3, Relational Operator3/1, Relational Operator2/1, Relational Operator/1
  OR/1 -> S-R Flip-Flop/2, S-R Flip-Flop1/2, HDL Counter1/1, HDL Counter/1
  start_bit_detected/1 -> S-R Flip-Flop1/1
  S-R Flip-Flop1/1 -> clk_start_bit_poll_cnt/2, Switch/2
  Constant/1 -> Switch/3
  Switch/1 -> HDL Counter1/2
  S-R Flip-Flop1/2 -> Terminator1/1
  Constant1/1 -> Relational Operator2/2
  Relational Operator2/1 -> clk_start_bit_poll_cnt/4, condition_for_start_sampling_position_data/1
  Constant2/1 -> Relational Operator3/2
  Relational Operator3/1 -> condition_for_sampling_the_error_bit/1

== system uz_endat_interface_2025b/uz_endat_interface/serial_communication/endat_clock_generator ==
  endat_clk_divider : Inport
  endat_clk_reset : Inport  Port=2
  endat_clk_enb : Inport  Port=3
  AND : Logic  IconShape=distinctive  AllPortsSameDT=off  OutDataTypeStr=boolean
  AND1 : Logic  IconShape=distinctive  AllPortsSameDT=off  OutDataTypeStr=boolean
  Constant : Constant  OutDataTypeStr=uint16  SampleTime=t_clock
  Data Type Conversion : DataTypeConversion  OutDataTypeStr=uint16  SaturateOnIntegerOverflow=off  RndMeth=Floor
  Delay : Delay  DelayLength=1
  Delay1 : Delay  DelayLength=1
  Detect Rise Positive1 : simulink/Logic and Bit Operations/Detect Rise Positive  vinit=0  OutDataTypeStr=boolean
  OR : Logic  Operator=OR  IconShape=distinctive  AllPortsSameDT=off  OutDataTypeStr=boolean
  Relational Operator : RelationalOperator  OutDataTypeStr=boolean  RndMeth=Simplest  InputSameDT=off
  S-R Flip-Flop1 : simulink_extras/Flip Flops/S-R Flip-Flop  initial_condition=0
  Sum : Sum  Inputs=|+-  AccumDataTypeStr=uint16
  base_counter : hdlsllib/Sources/HDL Counter  CountType=Free running  CountInit=0  CountStep=1  CountMax=199  CountFromType=Initial value  CountFrom=0  CountResetPort=on  CountLoadPort=off  CountEnbPort=on  CountDirPort=off  CountHitOutputPort=off  CountDataType=Unsigned  CountWordLen=16  CountFracLen=0  CountSampTime=1
  endat_clk : Outport
  wires:
  base_counter/1 -> Relational Operator/1, Detect Rise Positive1/1
  endat_clk_reset/1 -> OR/2
  Detect Rise Positive1/1 -> AND/1, AND1/2
  S-R Flip-Flop1/1 -> endat_clk/1, Delay/1
  S-R Flip-Flop1/2 -> Delay1/1
  Delay/1 -> AND/2
  Delay1/1 -> AND1/1
  AND/1 -> OR/1
  endat_clk_divider/1 -> Data Type Conversion/1
  Data Type Conversion/1 -> Sum/1
  Constant/1 -> Sum/2
  Sum/1 -> Relational Operator/2
  Relational Operator/1 -> base_counter/1
  AND1/1 -> S-R Flip-Flop1/1
  OR/1 -> S-R Flip-Flop1/2
  endat_clk_enb/1 -> base_counter/2

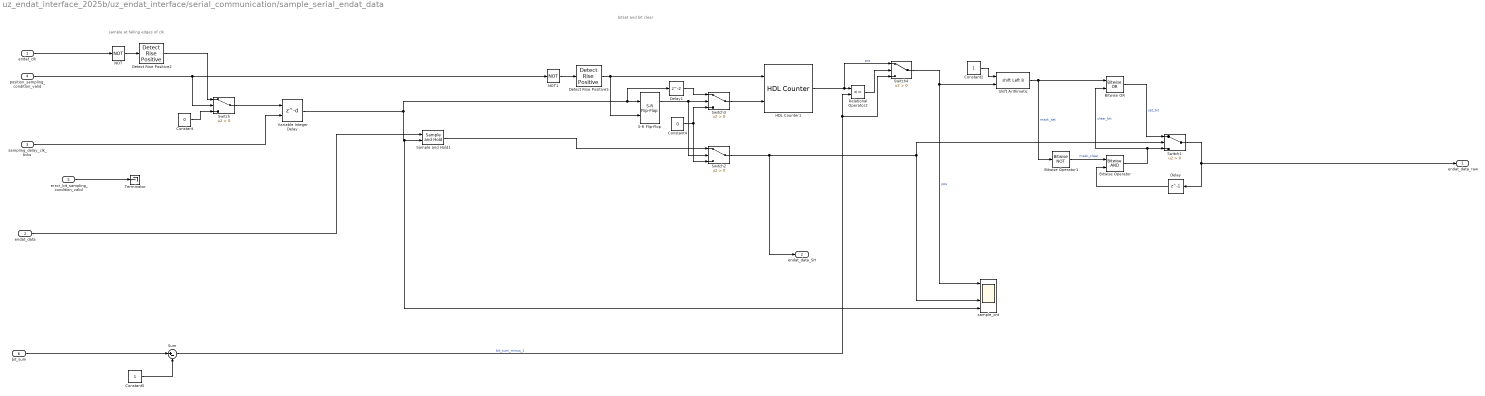
== system uz_endat_interface_2025b/uz_endat_interface/serial_communication/sample_serial_endat_data ==
  note: bitset and bit clear
  note: sample at falling edges of clk
  endat_clk : Inport
  endat_data : Inport  Port=2
  sampling_delay_clk_ticks : Inport  Port=3  OutDataTypeStr=uint32
  position_sampling_condition_valid : Inport  Port=4
  error_bit_sampling_condition_valid : Inport  Port=5
  bit_sum : Inport  Port=6
  Bitwise Operator : simulink/Logic and Bit Operations/Bitwise Operator  logicop=AND  UseBitMask=off  NumInputPorts=2  BitMask=bin2dec('11011001')  BitMaskRealWorld=Stored Integer
  Bitwise Operator1 : simulink/Logic and Bit Operations/Bitwise Operator  logicop=NOT  UseBitMask=off  BitMask=bin2dec('11011001')  BitMaskRealWorld=Stored Integer
  Bitwise OR : simulink/Logic and Bit Operations/Bitwise Operator  logicop=OR  UseBitMask=off  NumInputPorts=2  BitMask=bin2dec('11011001')  BitMaskRealWorld=Stored Integer
      settings: LibrarySourceBlock=|
      | simulink/Quick Insert/Logic and Bit
      | Operations/Bitwise OR
  Constant : Constant  Value=0  OutDataTypeStr=boolean  SampleTime=t_clock
  Constant2 : Constant  OutDataTypeStr=uint64  SampleTime=t_clock
  Constant4 : Constant  Value=0  OutDataTypeStr=boolean  SampleTime=t_clock
  Constant5 : Constant  OutDataTypeStr=uint32  SampleTime=-1
  Delay : Delay  DelayLength=1
  Delay1 : Delay
  Detect Rise Positive2 : simulink/Logic and Bit Operations/Detect Rise Positive  vinit=0  OutDataTypeStr=boolean
  Detect Rise Positive5 : simulink/Logic and Bit Operations/Detect Rise Positive  vinit=0  OutDataTypeStr=boolean
  HDL Counter1 : hdlsllib/Sources/HDL Counter  CountType=Free running  CountInit=0  CountStep=1  CountMax=24  CountFromType=Initial value  CountFrom=0  CountResetPort=on  CountLoadPort=off  CountEnbPort=on  CountDirPort=off  CountHitOutputPort=off  CountDataType=Unsigned  CountWordLen=6  CountFracLen=0  CountSampTime=1
  NOT : Logic  Operator=NOT  IconShape=distinctive  AllPortsSameDT=off  OutDataTypeStr=boolean
  NOT1 : Logic  Operator=NOT  IconShape=distinctive  AllPortsSameDT=off  OutDataTypeStr=boolean
  Relational Operator2 : RelationalOperator  Operator=<=  OutDataTypeStr=boolean  RndMeth=Simplest  InputSameDT=off
  S-R Flip-Flop : simulink_extras/Flip Flops/S-R Flip-Flop  initial_condition=0
  Sample and Hold1 : spsSampleandHoldLib/Sample and Hold  ic=0  Ts=t_clock
      settings: LibrarySourceBlock=|
      | sps_lib/Control/Sample and
      | Hold
  Shift Arithmetic : ArithShift  BitShiftNumberSource=Input port  BitShiftNumber=8  BitShiftDirection=Left
      settings: InputPortMap=u0,p1
  Sum : Sum  Inputs=|+-  OutDataTypeStr=uint32
  Switch{,1..4} (5 alike) : Switch  Criteria=u2 > Threshold  SaturateOnIntegerOverflow=off  InputSameDT=off
  Terminator : Terminator
  Variable Integer Delay : Delay  DelayLengthSource=Input port  SampleTime=t_clock
      settings: InputPortMap=u0,p1
  sample_cnt : Scope  NumInputPorts=4
      settings: ActiveDisplayYMinimum=-5.1249999999999991  ActiveDisplayYMaximum=46.125  DataLoggingVariableName=ScopeData6
  endat_data_raw : Outport  OutDataTypeStr=uint64
  endat_data_SH : Outport  Port=2
  wires:
  NOT/1 -> Detect Rise Positive2/1
  endat_data/1 -> Sample and Hold1/1
  position_sampling_condition_valid/1 -> NOT1/1, Switch/2
  Switch/1 -> Variable Integer Delay/1
  Constant/1 -> Switch/3
  endat_clk/1 -> NOT/1
  Switch4/1 -> sample_cnt/1, Shift Arithmetic/2  "pos"
  Constant2/1 -> Shift Arithmetic/1
  Shift Arithmetic/1 -> Bitwise OR/1, Bitwise Operator1/1  "mask_set"
  Bitwise OR/1 -> Switch1/1  "set_bit"
  Switch2/1 -> Switch1/2, sample_cnt/3, endat_data_SH/1
  Bitwise Operator1/1 -> Bitwise Operator/1  "mask_clear"
  Bitwise Operator/1 -> Switch1/3, Bitwise OR/2  "clear_bit"
  Delay/1 -> Bitwise Operator/2
  Switch1/1 -> endat_data_raw/1, Delay/1
  sampling_delay_clk_ticks/1 -> Variable Integer Delay/2
  error_bit_sampling_condition_valid/1 -> Terminator/1
  Constant5/1 -> Sum/2
  bit_sum/1 -> Sum/1
  Detect Rise Positive2/1 -> Switch/1
  NOT1/1 -> Detect Rise Positive5/1
  Detect Rise Positive5/1 -> S-R Flip-Flop/2, HDL Counter1/1
  Variable Integer Delay/1 -> sample_cnt/4, Sample and Hold1/2, Delay1/1, S-R Flip-Flop/1
  S-R Flip-Flop/1 -> Switch2/2, Switch3/2
  Switch3/1 -> HDL Counter1/2
  Delay1/1 -> Switch3/1
  Constant4/1 -> Switch2/3, Switch3/3
  Sample and Hold1/1 -> Switch2/1
  HDL Counter1/1 -> Switch4/1, Relational Operator2/1  "pos"
  Relational Operator2/1 -> Switch4/2
  Sum/1 -> Switch4/3, Relational Operator2/2  "bit_sum_minus_1"

== system uz_endat_interface_2025b/uz_endat_interface/set_offset_to_raw_position_and_wrap/floor_div_pow2 ==
  note: This is a integer divison for a int64 dividend that is divided by a divisor which is a power of two (2^n) with rounding mode 'floor' of the result.
      | The Simulink divide block offers the same calculation but is not supported by the HDL-Coder in rounding mode 'floor'. Therefore, this is a manually built version made from basic operations.
  dividend : Inport
  divisor_power_of_two_bits : Inport  Port=2
  AND2 : Logic  IconShape=distinctive  AllPortsSameDT=off  OutDataTypeStr=boolean
  Bitwise AND6 : simulink/Logic and Bit Operations/Bitwise Operator  logicop=AND  UseBitMask=off  NumInputPorts=2  BitMask=bin2dec('11011001')  BitMaskRealWorld=Stored Integer
      settings: LibrarySourceBlock=|
      | simulink/Quick Insert/Logic and Bit
      | Operations/Bitwise AND
  Constant : Constant  Value=0  OutDataTypeStr=int64  SampleTime=-1
  Relational Operator : RelationalOperator  Operator=<  OutDataTypeStr=boolean  RndMeth=Simplest  InputSameDT=off
  Relational Operator1 : RelationalOperator  Operator=~=  OutDataTypeStr=boolean  RndMeth=Simplest  InputSameDT=off
  Shift Arithmetic4 : ArithShift  BitShiftNumberSource=Input port  BitShiftNumber=8  BitShiftDirection=Right
      settings: InputPortMap=u0,p1
  Shift Arithmetic5 : ArithShift  BitShiftNumberSource=Input port  BitShiftNumber=8  BitShiftDirection=Left
      settings: InputPortMap=u0,p1
  Sum10 : Sum  Inputs=|+-  OutDataTypeStr=int64
  Sum9 : Sum  Inputs=|+-  OutDataTypeStr=int64
  Switch : Switch  Criteria=u2 > Threshold  SaturateOnIntegerOverflow=off  InputSameDT=off
  const4 : Constant  OutDataTypeStr=int64  SampleTime=t_clock
  quotient : Outport
  wires:
  const4/1 -> Sum10/2, Sum9/2, Shift Arithmetic5/1
  Relational Operator1/1 -> AND2/2
  Relational Operator/1 -> AND2/1
  Switch/1 -> quotient/1  "quotient"
  Bitwise AND6/1 -> Relational Operator1/1  "rem_bits"
  Sum10/1 -> Switch/1  "q_trunc minus one"
  dividend/1 -> Relational Operator/1, Bitwise AND6/1, Shift Arithmetic4/1
  Shift Arithmetic4/1 -> Sum10/1, Switch/3  "q_trunc"
  Shift Arithmetic5/1 -> Sum9/1
  divisor_power_of_two_bits/1 -> Shift Arithmetic4/2, Shift Arithmetic5/2
  Sum9/1 -> Bitwise AND6/2  "mask"
  AND2/1 -> Switch/2
  Constant/1 -> Relational Operator/2, Relational Operator1/2

== matlab function uz_endat_interface_2025b/endat_encoder_Heidenhain_MT12bit_ST25bit/create_ST_and_MT_position_values/MATLAB Function ==
  data: u input; y output
function y = BinaryToGray(u)
%#codegen

y = bitxor(u,(bitshift(u,-1)));

== matlab function uz_endat_interface_2025b/uz_endat_interface/wrap_2pi/fixed_point_floor ==
  settings: fimath=fimath('RoundingMethod', 'Floor','OverflowAction', 'Wrap','ProductMode', 'FullPrecision', 'SumMode', 'FullPrecision')
  data: x input; y output
function y = fcn(x)
%#codegen
x_floor = bitsra(x, x.FractionLength);  % Shift right to remove fraction
x_floor = bitsll(x_floor, x.FractionLength);  % Shift left to restore scale

y = x_floor;

== matlab function uz_endat_interface_2025b/uz_endat_interface/position_to_speed_pll/fixed_point_floor ==
  settings: fimath=fimath('RoundingMethod', 'Floor','OverflowAction', 'Wrap','ProductMode', 'FullPrecision', 'SumMode', 'FullPrecision')
  data: x input; y output
function y = fcn(x)
%#codegen
x_floor = bitsra(x, x.FractionLength);  % Shift right to remove fraction
x_floor = bitsll(x_floor, x.FractionLength);  % Shift left to restore scale

y = x_floor;

== matlab function uz_endat_interface_2025b/endat_encoder_Heidenhain_MT12bit_ST25bit/create_ST_and_MT_position_values/MATLAB Function1 ==
  data: u input; y output
function y = reverseBits(u)
%#codegen
% Reverse bit order for an unsigned fixed-point input (ufixN)

    % Determine word length from type
    BW = numerictype(u).WordLength;

    % Prepare output with same numerictype
    y = fi(0, numerictype(u), fimath(u));

    tmp = u;

    % Bit-by-bit reversal
    for i = 0:(BW-1)
        % Extract LSB, shift to MSB side, OR accumulate
        y = bitor(y, bitshift(bitand(tmp, fi(1, numerictype(u))), BW-1-i));
        tmp = bitshift(tmp, -1);
    end
end

== matlab function uz_endat_interface_2025b/endat_encoder_Heidenhain_MT12bit_ST25bit/create_ST_and_MT_position_values/MATLAB Function2 ==
  data: u input; y output
function y = reverseBits(u)
%#codegen
% Reverse bit order for an unsigned fixed-point input (ufixN)

    % Determine word length from type
    BW = numerictype(u).WordLength;

    % Prepare output with same numerictype
    y = fi(0, numerictype(u), fimath(u));

    tmp = u;

    % Bit-by-bit reversal
    for i = 0:(BW-1)
        % Extract LSB, shift to MSB side, OR accumulate
        y = bitor(y, bitshift(bitand(tmp, fi(1, numerictype(u))), BW-1-i));
        tmp = bitshift(tmp, -1);
    end
end
